simulink model "model_static_wind_field"  (R2020b)
settings: configuration reference "Configuration" (kept outside this file)
undefined symbols (not defined in the file or in its folder): HEIGHT_BREAKPOINTS, hours_u, hours_v, hours_w, lat_breakpoints, lon_breakpoints, matrix_idx
settings Model: Creator=Dogukan  LastModifiedBy=dogukan
settings ConfigSetRef: SourceName=Configuration  SourceLocation=Base Workspace

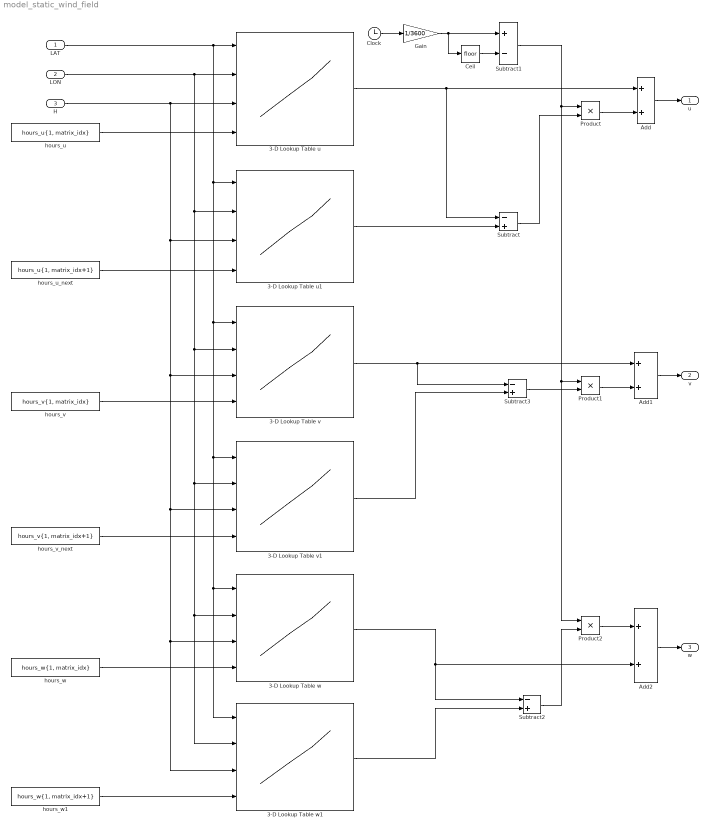
== system model_static_wind_field ==
  LAT : Inport
  LON : Inport  Port=2
  H : Inport  Port=3
  3-D Lookup Table u : Lookup_n-D  NumberOfTableDimensions=3  BreakpointsForDimension1=lat_breakpoints  BreakpointsForDimension2=lon_breakpoints  BreakpointsForDimension3=flip(HEIGHT_BREAKPOINTS)  TableSource=Input port  Table=hours_u{1, 1}  ExtrapMethod=Clip  InternalRulePriority=Speed  RndMeth=Simplest  InputSameDT=on
      settings: InputPortMap=u0,u1,u2,p221
  3-D Lookup Table u1 : Lookup_n-D  NumberOfTableDimensions=3  BreakpointsForDimension1=lat_breakpoints  BreakpointsForDimension2=lon_breakpoints  BreakpointsForDimension3=flip(HEIGHT_BREAKPOINTS)  TableSource=Input port  Table=hours_u{1, 1}  ExtrapMethod=Clip  InternalRulePriority=Speed  RndMeth=Simplest  InputSameDT=on
      settings: InputPortMap=u0,u1,u2,p221
  3-D Lookup Table v : Lookup_n-D  NumberOfTableDimensions=3  BreakpointsForDimension1=lat_breakpoints  BreakpointsForDimension2=lon_breakpoints  BreakpointsForDimension3=flip(HEIGHT_BREAKPOINTS)  TableSource=Input port  Table=reshape(repmat([4 5 6;16 19 20;10 18 23],1,2),[3,3,2])  ExtrapMethod=Clip  InternalRulePriority=Speed  RndMeth=Simplest  InputSameDT=on
      settings: InputPortMap=u0,u1,u2,p221
  3-D Lookup Table v1 : Lookup_n-D  NumberOfTableDimensions=3  BreakpointsForDimension1=lat_breakpoints  BreakpointsForDimension2=lon_breakpoints  BreakpointsForDimension3=flip(HEIGHT_BREAKPOINTS)  TableSource=Input port  Table=reshape(repmat([4 5 6;16 19 20;10 18 23],1,2),[3,3,2])  ExtrapMethod=Clip  InternalRulePriority=Speed  RndMeth=Simplest  InputSameDT=on
      settings: InputPortMap=u0,u1,u2,p221
  3-D Lookup Table w : Lookup_n-D  NumberOfTableDimensions=3  BreakpointsForDimension1=lat_breakpoints  BreakpointsForDimension2=lon_breakpoints  BreakpointsForDimension3=flip(HEIGHT_BREAKPOINTS)  TableSource=Input port  Table=reshape(repmat([4 5 6;16 19 20;10 18 23],1,2),[3,3,2])  ExtrapMethod=Clip  InternalRulePriority=Speed  RndMeth=Simplest  InputSameDT=on
      settings: InputPortMap=u0,u1,u2,p221
  3-D Lookup Table w1 : Lookup_n-D  NumberOfTableDimensions=3  BreakpointsForDimension1=lat_breakpoints  BreakpointsForDimension2=lon_breakpoints  BreakpointsForDimension3=flip(HEIGHT_BREAKPOINTS)  TableSource=Input port  Table=reshape(repmat([4 5 6;16 19 20;10 18 23],1,2),[3,3,2])  ExtrapMethod=Clip  InternalRulePriority=Speed  RndMeth=Simplest  InputSameDT=on
      settings: InputPortMap=u0,u1,u2,p221
  Add : Sum
  Add1 : Sum
  Add2 : Sum
  Ceil : Rounding
  Clock : Clock
  Gain : Gain  Gain=1/3600
  Product : Product
  Product1 : Product
  Product2 : Product
  Subtract : Sum  Inputs=-+
  Subtract1 : Sum  Inputs=+-
  Subtract2 : Sum  Inputs=-+
  Subtract3 : Sum  Inputs=-+
  hours_u : Constant  Value=hours_u{1, matrix_idx}  OutDataTypeStr=single
  hours_u_next : Constant  Value=hours_u{1, matrix_idx+1}  OutDataTypeStr=single
  hours_v : Constant  Value=hours_v{1, matrix_idx}
  hours_v_next : Constant  Value=hours_v{1, matrix_idx+1}
  hours_w : Constant  Value=hours_w{1, matrix_idx}
  hours_w1 : Constant  Value=hours_w{1, matrix_idx+1}
  u : Outport  SignalName=u
  v : Outport  Port=2  SignalName=v
  w : Outport  Port=3  SignalName=w
  wires:
  LAT/1 -> 3-D Lookup Table u/1, 3-D Lookup Table u1/1, 3-D Lookup Table v1/1, 3-D Lookup Table w1/1, 3-D Lookup Table w/1, 3-D Lookup Table v/1
  LON/1 -> 3-D Lookup Table u1/2, 3-D Lookup Table v1/2, 3-D Lookup Table w1/2, 3-D Lookup Table w/2, 3-D Lookup Table v/2, 3-D Lookup Table u/2
  H/1 -> 3-D Lookup Table u1/3, 3-D Lookup Table v1/3, 3-D Lookup Table w1/3, 3-D Lookup Table w/3, 3-D Lookup Table v/3, 3-D Lookup Table u/3
  3-D Lookup Table u/1 -> Add/1, Subtract/1
  hours_w/1 -> 3-D Lookup Table w/4
  hours_v/1 -> 3-D Lookup Table v/4
  hours_u/1 -> 3-D Lookup Table u/4
  hours_u_next/1 -> 3-D Lookup Table u1/4
  Clock/1 -> Gain/1
  Gain/1 -> Ceil/1, Subtract1/1
  3-D Lookup Table u1/1 -> Subtract/2
  Subtract/1 -> Product/2
  Product/1 -> Add/2
  Ceil/1 -> Subtract1/2
  Subtract1/1 -> Product2/1, Product1/1, Product/1
  Add/1 -> u/1
  hours_v_next/1 -> 3-D Lookup Table v1/4
  3-D Lookup Table v/1 -> Add1/1, Subtract3/1
  3-D Lookup Table v1/1 -> Subtract3/2
  Add1/1 -> v/1
  Subtract3/1 -> Product1/2
  Product1/1 -> Add1/2
  hours_w1/1 -> 3-D Lookup Table w1/4
  3-D Lookup Table w/1 -> Subtract2/1, Add2/2
  Add2/1 -> w/1
  Subtract2/1 -> Product2/2
  3-D Lookup Table w1/1 -> Subtract2/2
  Product2/1 -> Add2/1
